simulink model "w3_warplab_trigger_proc"  (Simulink 7.7)
settings: Solver=ode45  StartTime=0.0  StopTime=60  RelTol=1e-3
InitFcn:
  | w3_warplab_trigger_proc_init
StartFcn:
  | w3_warplab_trigger_proc_init
undefined symbols (not defined in the file): gcbh, xlBlockLoadCallback, xlGetNormalizedPeriod
libraries: xbsIndex_r4 x1289, xbsEDKLib_r4 x1, simulink x1
(part 7 of 10)

== system w3_warplab_trigger_proc/Trigger Sources/CM PLL 2 ==
  Debounce Register{1..4} (4 alike) : xbsIndex_r4/Register  init=0  rst=off  en=off  dbl_ovrd=off  block_type=register
  Logical : xbsIndex_r4/Logical  logical_function=AND  inputs=4  en=off  latency=0  precision=Full  arith_type=Unsigned  n_bits=16  bin_pt=0  align_bp=on  dbl_ovrd=off  block_type=logical
  Mux : xbsIndex_r4/Mux  inputs=2  en=off  latency=0  precision=Full  arith_type=Unsigned  n_bits=16  bin_pt=14  quantization=Truncate  overflow=Wrap  dbl_ovrd=off  block_type=mux
  Trigger : Outport
  wires:
  Mux/1 -> Trigger/1
  Debounce Register1/1 -> Debounce Register2/1, Logical/1
  Debounce Register2/1 -> Debounce Register3/1, Logical/2
  Debounce Register3/1 -> Debounce Register4/1, Logical/3
  [Debug_2_Debounce] -> Mux/1
  Debounce Register4/1 -> Logical/4
  Logical/1 -> Mux/3
  [TRIG_DELAYED_CM_PLL_2] -> Mux/2, Debounce Register1/1

== system w3_warplab_trigger_proc/Trigger Sources/CM PLL 3 ==
  Debounce Register{1..4} (4 alike) : xbsIndex_r4/Register  init=0  rst=off  en=off  dbl_ovrd=off  block_type=register
  Logical : xbsIndex_r4/Logical  logical_function=AND  inputs=4  en=off  latency=0  precision=Full  arith_type=Unsigned  n_bits=16  bin_pt=0  align_bp=on  dbl_ovrd=off  block_type=logical
  Mux : xbsIndex_r4/Mux  inputs=2  en=off  latency=0  precision=Full  arith_type=Unsigned  n_bits=16  bin_pt=14  quantization=Truncate  overflow=Wrap  dbl_ovrd=off  block_type=mux
  Trigger : Outport
  wires:
  Logical/1 -> Mux/3
  Debounce Register4/1 -> Logical/4
  [Debug_3_Debounce] -> Mux/1
  Debounce Register3/1 -> Logical/3, Debounce Register4/1
  Debounce Register2/1 -> Logical/2, Debounce Register3/1
  Debounce Register1/1 -> Logical/1, Debounce Register2/1
  Mux/1 -> Trigger/1
  [TRIG_DELAYED_CM_PLL_3] -> Debounce Register1/1, Mux/2

== system w3_warplab_trigger_proc/Trigger Sources/Debug 0 ==
  Debounce Register{1..4} (4 alike) : xbsIndex_r4/Register  init=0  rst=off  en=off  dbl_ovrd=off  block_type=register
  Logical : xbsIndex_r4/Logical  logical_function=AND  inputs=4  en=off  latency=0  precision=Full  arith_type=Unsigned  n_bits=16  bin_pt=0  align_bp=on  dbl_ovrd=off  block_type=logical
  Mux : xbsIndex_r4/Mux  inputs=2  en=off  latency=0  precision=Full  arith_type=Unsigned  n_bits=16  bin_pt=14  quantization=Truncate  overflow=Wrap  dbl_ovrd=off  block_type=mux
  Trigger : Outport
  wires:
  Mux/1 -> Trigger/1
  Debounce Register1/1 -> Debounce Register2/1, Logical/1
  Debounce Register2/1 -> Logical/2, Debounce Register3/1
  Debounce Register3/1 -> Debounce Register4/1, Logical/3
  [Debug_0_Debounce] -> Mux/1
  Debounce Register4/1 -> Logical/4
  Logical/1 -> Mux/3
  [TRIG_DELAYED_DBG_HDR_0] -> Mux/2, Debounce Register1/1

== system w3_warplab_trigger_proc/Trigger Sources/Debug 1 ==
  Debounce Register{1..4} (4 alike) : xbsIndex_r4/Register  init=0  rst=off  en=off  dbl_ovrd=off  block_type=register
  Logical : xbsIndex_r4/Logical  logical_function=AND  inputs=4  en=off  latency=0  precision=Full  arith_type=Unsigned  n_bits=16  bin_pt=0  align_bp=on  dbl_ovrd=off  block_type=logical
  Mux : xbsIndex_r4/Mux  inputs=2  en=off  latency=0  precision=Full  arith_type=Unsigned  n_bits=16  bin_pt=14  quantization=Truncate  overflow=Wrap  dbl_ovrd=off  block_type=mux
  Trigger : Outport
  wires:
  Logical/1 -> Mux/3
  Debounce Register4/1 -> Logical/4
  [Debug_1_Debounce] -> Mux/1
  Debounce Register3/1 -> Logical/3, Debounce Register4/1
  Debounce Register2/1 -> Logical/2, Debounce Register3/1
  Debounce Register1/1 -> Logical/1, Debounce Register2/1
  Mux/1 -> Trigger/1
  [TRIG_DELAYED_DBG_HDR_1] -> Debounce Register1/1, Mux/2

== system w3_warplab_trigger_proc/Trigger Sources/Debug 2 ==
  Debounce Register{1..4} (4 alike) : xbsIndex_r4/Register  init=0  rst=off  en=off  dbl_ovrd=off  block_type=register
  Logical : xbsIndex_r4/Logical  logical_function=AND  inputs=4  en=off  latency=0  precision=Full  arith_type=Unsigned  n_bits=16  bin_pt=0  align_bp=on  dbl_ovrd=off  block_type=logical
  Mux : xbsIndex_r4/Mux  inputs=2  en=off  latency=0  precision=Full  arith_type=Unsigned  n_bits=16  bin_pt=14  quantization=Truncate  overflow=Wrap  dbl_ovrd=off  block_type=mux
  Trigger : Outport
  wires:
  Mux/1 -> Trigger/1
  Debounce Register1/1 -> Debounce Register2/1, Logical/1
  Debounce Register2/1 -> Debounce Register3/1, Logical/2
  Debounce Register3/1 -> Debounce Register4/1, Logical/3
  [Debug_2_Debounce] -> Mux/1
  Debounce Register4/1 -> Logical/4
  Logical/1 -> Mux/3
  [TRIG_DELAYED_DBG_HDR_2] -> Mux/2, Debounce Register1/1

== system w3_warplab_trigger_proc/Trigger Sources/Debug 3 ==
  Debounce Register{1..4} (4 alike) : xbsIndex_r4/Register  init=0  rst=off  en=off  dbl_ovrd=off  block_type=register
  Logical : xbsIndex_r4/Logical  logical_function=AND  inputs=4  en=off  latency=0  precision=Full  arith_type=Unsigned  n_bits=16  bin_pt=0  align_bp=on  dbl_ovrd=off  block_type=logical
  Mux : xbsIndex_r4/Mux  inputs=2  en=off  latency=0  precision=Full  arith_type=Unsigned  n_bits=16  bin_pt=14  quantization=Truncate  overflow=Wrap  dbl_ovrd=off  block_type=mux
  Trigger : Outport
  wires:
  Logical/1 -> Mux/3
  Debounce Register4/1 -> Logical/4
  [Debug_3_Debounce] -> Mux/1
  Debounce Register3/1 -> Logical/3, Debounce Register4/1
  Debounce Register2/1 -> Logical/2, Debounce Register3/1
  Debounce Register1/1 -> Logical/1, Debounce Register2/1
  Mux/1 -> Trigger/1
  [TRIG_DELAYED_DBG_HDR_3] -> Debounce Register1/1, Mux/2

== system w3_warplab_trigger_proc/Trigger Sources/Energy ==
  16LSB : xbsIndex_r4/Slice  nbits=16  boolean_output=off  mode=Lower Bit Location + Width  bit1=0  base1=MSB of Input  bit0=0  base0=LSB of Input  dbl_ovrd=off  block_type=slice
  16MSB : xbsIndex_r4/Slice  nbits=16  boolean_output=off  mode=Lower Bit Location + Width  bit1=0  base1=MSB of Input  bit0=16  base0=LSB of Input  dbl_ovrd=off  block_type=slice
  AntA Detector : Subsystem
  AntB Detector : Subsystem
  AntC Detector : Subsystem
  AntD Detector : Subsystem
  Convert : xbsIndex_r4/Convert  gui_display_data_type=Boolean  arith_type=Boolean  n_bits=16  bin_pt=14  float_type=Single  exp_bits=8  fraction_bits=24  quantization=Truncate  overflow=Wrap  en=off  latency=0  dbl_ovrd=off  pipeline=off  block_type=convert
  Display : Display
      settings: Format=hex (Stored Integer)
  Display1 : Display
      settings: Format=hex (Stored Integer)
  Display2 : Display
      settings: Format=hex (Stored Integer)
  Gateway Out1 : xbsIndex_r4/Gateway Out  inherit_from_input=off  hdl_port=off  timing_constraint=None  locs_specified=off  LOCs={}  UseAsDAC=off  DACChannel='1'  block_type=gatewayout
  Gateway Out2 : xbsIndex_r4/Gateway Out  inherit_from_input=off  hdl_port=off  timing_constraint=None  locs_specified=off  LOCs={}  UseAsDAC=off  DACChannel='1'  block_type=gatewayout
  Gateway Out6 : xbsIndex_r4/Gateway Out  inherit_from_input=off  hdl_port=off  timing_constraint=None  locs_specified=off  LOCs={}  UseAsDAC=off  DACChannel='1'  block_type=gatewayout
  MIMO Logic : Subsystem
  Posedge : Subsystem
  Pulse Generator : DiscretePulseGenerator  PulseType=Time based  Period=16  PulseWidth=50
  RFA_RSSI : xbsIndex_r4/Gateway In  gui_display_data_type=Fixed-point  arith_type=Unsigned  n_bits=10  bin_pt=0  preci_type=Single  exp_width=8  frac_width=24  quantization=Truncate  overflow=Wrap  period=1  dbl_ovrd=off  timing_constraint=None  locs_specified=off  LOCs={}  UseAsADC=off  ADCChannel='1'  inherit_from_input=off  hdl_port=on  block_type=gatewayin
      settings: block_version=VER_STRING_GOES_HERE
  RFB_RSSI : xbsIndex_r4/Gateway In  gui_display_data_type=Fixed-point  arith_type=Unsigned  n_bits=10  bin_pt=0  preci_type=Single  exp_width=8  frac_width=24  quantization=Truncate  overflow=Wrap  period=1  dbl_ovrd=off  timing_constraint=None  locs_specified=off  LOCs={}  UseAsADC=off  ADCChannel='1'  inherit_from_input=off  hdl_port=on  block_type=gatewayin
      settings: infoedit="Gateway in block.  Converts inputs of type Simulink integer, double and fixed point to  Xilinx fixed point type.<P><P>Hardware notes:  In hardware these blocks become top level input ports."  block_version=VER_STRING_GOES_HERE
  RFC_RSSI : xbsIndex_r4/Gateway In  gui_display_data_type=Fixed-point  arith_type=Unsigned  n_bits=10  bin_pt=0  preci_type=Single  exp_width=8  frac_width=24  quantization=Truncate  overflow=Wrap  period=1  dbl_ovrd=off  timing_constraint=None  locs_specified=off  LOCs={}  UseAsADC=off  ADCChannel='1'  inherit_from_input=off  hdl_port=on  block_type=gatewayin
      settings: infoedit="Gateway in block.  Converts inputs of type Simulink integer, double and fixed point to  Xilinx fixed point type.<P><P>Hardware notes:  In hardware these blocks become top level input ports."  block_version=VER_STRING_GOES_HERE
  RFD_RSSI : xbsIndex_r4/Gateway In  gui_display_data_type=Fixed-point  arith_type=Unsigned  n_bits=10  bin_pt=0  preci_type=Single  exp_width=8  frac_width=24  quantization=Truncate  overflow=Wrap  period=1  dbl_ovrd=off  timing_constraint=None  locs_specified=off  LOCs={}  UseAsADC=off  ADCChannel='1'  inherit_from_input=off  hdl_port=on  block_type=gatewayin
      settings: infoedit="Gateway in block.  Converts inputs of type Simulink integer, double and fixed point to  Xilinx fixed point type.<P><P>Hardware notes:  In hardware these blocks become top level input ports."  block_version=VER_STRING_GOES_HERE
  RSSI_CLK : xbsIndex_r4/Gateway In  gui_display_data_type=Boolean  arith_type=Boolean  n_bits=10  bin_pt=0  preci_type=Single  exp_width=8  frac_width=24  quantization=Truncate  overflow=Wrap  period=1  dbl_ovrd=off  timing_constraint=None  locs_specified=off  LOCs={}  UseAsADC=off  ADCChannel='1'  inherit_from_input=off  hdl_port=on  block_type=gatewayin
      settings: block_version=VER_STRING_GOES_HERE
  Repeating Sequence : simulink/Sources/Repeating Sequence  SystemSampleTime=-1  rep_seq_t=[0 200 600]  rep_seq_y=[0 1023 0]
  b0 : xbsIndex_r4/Slice  nbits=1  boolean_output=off  mode=Lower Bit Location + Width  bit1=0  base1=MSB of Input  bit0=0  base0=LSB of Input  dbl_ovrd=off  block_type=slice
  b1 : xbsIndex_r4/Slice  nbits=1  boolean_output=off  mode=Lower Bit Location + Width  bit1=0  base1=MSB of Input  bit0=1  base0=LSB of Input  dbl_ovrd=off  block_type=slice
  b2 : xbsIndex_r4/Slice  nbits=1  boolean_output=off  mode=Lower Bit Location + Width  bit1=0  base1=MSB of Input  bit0=2  base0=LSB of Input  dbl_ovrd=off  block_type=slice
  b3 : xbsIndex_r4/Slice  nbits=1  boolean_output=off  mode=Lower Bit Location + Width  bit1=0  base1=MSB of Input  bit0=3  base0=LSB of Input  dbl_ovrd=off  block_type=slice
  b31 : xbsIndex_r4/Slice  nbits=1  boolean_output=off  mode=Lower Bit Location + Width  bit1=0  base1=MSB of Input  bit0=31  base0=LSB of Input  dbl_ovrd=off  block_type=slice
  b[15:8] : xbsIndex_r4/Slice  nbits=8  boolean_output=off  mode=Lower Bit Location + Width  bit1=0  base1=MSB of Input  bit0=8  base0=LSB of Input  dbl_ovrd=off  block_type=slice
  b[20:16] : xbsIndex_r4/Slice  nbits=5  boolean_output=off  mode=Lower Bit Location + Width  bit1=0  base1=MSB of Input  bit0=16  base0=LSB of Input  dbl_ovrd=off  block_type=slice
  b[7:0] : xbsIndex_r4/Slice  nbits=8  boolean_output=off  mode=Lower Bit Location + Width  bit1=0  base1=MSB of Input  bit0=0  base0=LSB of Input  dbl_ovrd=off  block_type=slice
  Trigger : Outport
  tag scope: pktDetMask_A=global, pktDetMask_B=global, pktDetMask_C=global, pktDetMask_D=global, pktDetReset=global, pktDet_duration_busy=global, pktDet_duration_idle=global, pktDet_energyThresh_busy=global, pktDet_energyThresh_idle=global, regPktDet_RSSIavgLength=global
  wires:
  AntA Detector/1(pktdet) -> MIMO Logic/1(Det A)
  [pktDetReset] -> Convert/1
  RFA_RSSI/1 -> AntA Detector/1(RSSI)
  [reg_pkt_det_config] -> b0/1, b1/1, b2/1, b3/1, Gateway Out6/1, b31/1
  [reg_pkt_det_thresh] -> 16LSB/1, 16MSB/1, Gateway Out1/1
  [reg_pkt_det_duration] -> b[7:0]/1, b[15:8]/1, b[20:16]/1, Gateway Out2/1
  16LSB/1 -> [pktDet_energyThresh_idle]
  16MSB/1 -> [pktDet_energyThresh_busy]
  b[7:0]/1 -> [pktDet_duration_idle]
  b[15:8]/1 -> [pktDet_duration_busy]
  b[20:16]/1 -> [regPktDet_RSSIavgLength]
  AntB Detector/1(pktdet) -> MIMO Logic/2(Det B)
  AntC Detector/1(pktdet) -> MIMO Logic/3(Det C)
  AntD Detector/1(pktdet) -> MIMO Logic/4(Det D)
  RFB_RSSI/1 -> AntB Detector/1(RSSI)
  RFC_RSSI/1 -> AntC Detector/1(RSSI)
  RFD_RSSI/1 -> AntD Detector/1(RSSI)
  Convert/1 -> AntA Detector/2(Reset), AntB Detector/2(Reset), AntC Detector/2(Reset), AntD Detector/2(Reset)
  MIMO Logic/1(PktDet) -> Trigger/1
  RSSI_CLK/1 -> Posedge/1(D)
  Posedge/1(Q) -> AntC Detector/3(En), AntD Detector/3(En), AntB Detector/3(En), AntA Detector/3(En)
  Repeating Sequence/1 -> RFA_RSSI/1, RFB_RSSI/1, RFC_RSSI/1, RFD_RSSI/1
  Pulse Generator/1 -> RSSI_CLK/1
  Gateway Out6/1 -> Display/1
  Gateway Out1/1 -> Display1/1
  Gateway Out2/1 -> Display2/1
  b0/1 -> [pktDetMask_A]
  b1/1 -> [pktDetMask_B]
  b2/1 -> [pktDetMask_C]
  b3/1 -> [pktDetMask_D]
  b31/1 -> [pktDetReset]

== system w3_warplab_trigger_proc/Trigger Sources/Ethernet A ==
  Constant{,1..4,6..7} (7 alike) : Constant  Value=0
  ETH_A_AXI_STR_TDATA : xbsIndex_r4/Gateway In  gui_display_data_type=Fixed-point  arith_type=Unsigned  n_bits=32  bin_pt=0  preci_type=Single  exp_width=8  frac_width=24  quantization="Round  (unbiased: +/- Inf)"  overflow=Wrap  period=1  dbl_ovrd=off  timing_constraint=None  locs_specified=off  LOCs={}  UseAsADC=off  ADCChannel='1'  inherit_from_input=off  hdl_port=on  block_type=gatewayin
  ETH_A_AXI_STR_TDEST : xbsIndex_r4/Gateway In  gui_display_data_type=Fixed-point  arith_type=Unsigned  n_bits=4  bin_pt=0  preci_type=Single  exp_width=8  frac_width=24  quantization="Round  (unbiased: +/- Inf)"  overflow=Wrap  period=1  dbl_ovrd=off  timing_constraint=None  locs_specified=off  LOCs={}  UseAsADC=off  ADCChannel='1'  inherit_from_input=off  hdl_port=on  block_type=gatewayin
  ETH_A_AXI_STR_TKEEP : xbsIndex_r4/Gateway In  gui_display_data_type=Fixed-point  arith_type=Unsigned  n_bits=4  bin_pt=0  preci_type=Single  exp_width=8  frac_width=24  quantization="Round  (unbiased: +/- Inf)"  overflow=Wrap  period=1  dbl_ovrd=off  timing_constraint=None  locs_specified=off  LOCs={}  UseAsADC=off  ADCChannel='1'  inherit_from_input=off  hdl_port=on  block_type=gatewayin
  ETH_A_AXI_STR_TLAST : xbsIndex_r4/Gateway In  gui_display_data_type=Fixed-point  arith_type=Unsigned  n_bits=1  bin_pt=0  preci_type=Single  exp_width=8  frac_width=24  quantization="Round  (unbiased: +/- Inf)"  overflow=Wrap  period=1  dbl_ovrd=off  timing_constraint=None  locs_specified=off  LOCs={}  UseAsADC=off  ADCChannel='1'  inherit_from_input=off  hdl_port=on  block_type=gatewayin
  ETH_A_AXI_STR_TREADY : xbsIndex_r4/Gateway In  gui_display_data_type=Fixed-point  arith_type=Unsigned  n_bits=1  bin_pt=0  preci_type=Single  exp_width=8  frac_width=24  quantization="Round  (unbiased: +/- Inf)"  overflow=Wrap  period=1  dbl_ovrd=off  timing_constraint=None  locs_specified=off  LOCs={}  UseAsADC=off  ADCChannel='1'  inherit_from_input=off  hdl_port=on  block_type=gatewayin
  ETH_A_AXI_STR_TSTRB : xbsIndex_r4/Gateway In  gui_display_data_type=Fixed-point  arith_type=Unsigned  n_bits=4  bin_pt=0  preci_type=Single  exp_width=8  frac_width=24  quantization="Round  (unbiased: +/- Inf)"  overflow=Wrap  period=1  dbl_ovrd=off  timing_constraint=None  locs_specified=off  LOCs={}  UseAsADC=off  ADCChannel='1'  inherit_from_input=off  hdl_port=on  block_type=gatewayin
  ETH_A_AXI_STR_TVALID : xbsIndex_r4/Gateway In  gui_display_data_type=Fixed-point  arith_type=Unsigned  n_bits=1  bin_pt=0  preci_type=Single  exp_width=8  frac_width=24  quantization="Round  (unbiased: +/- Inf)"  overflow=Wrap  period=1  dbl_ovrd=off  timing_constraint=None  locs_specified=off  LOCs={}  UseAsADC=off  ADCChannel='1'  inherit_from_input=off  hdl_port=on  block_type=gatewayin
  HW_SW_Select : xbsIndex_r4/Mux  inputs=2  en=off  latency=0  precision=Full  arith_type=Unsigned  n_bits=16  bin_pt=14  quantization=Truncate  overflow=Wrap  dbl_ovrd=off  block_type=mux
  Pkt Comp : Subsystem
  Terminator : Terminator
  Terminator1 : Terminator
  Terminator2 : Terminator
  Trigger : Outport
  wires:
  Constant/1 -> ETH_A_AXI_STR_TVALID/1
  Constant1/1 -> ETH_A_AXI_STR_TDATA/1
  Constant2/1 -> ETH_A_AXI_STR_TLAST/1
  Constant3/1 -> ETH_A_AXI_STR_TSTRB/1
  ETH_A_AXI_STR_TVALID/1 -> Pkt Comp/1(TVALID)  "TVALID"
  ETH_A_AXI_STR_TDATA/1 -> Pkt Comp/2(TDATA)  "TDATA"
  ETH_A_AXI_STR_TREADY/1 -> Pkt Comp/3(TREADY)  "TREADY"
  Constant4/1 -> ETH_A_AXI_STR_TREADY/1
  ETH_A_AXI_STR_TLAST/1 -> Pkt Comp/4(TLAST)  "TLAST"
  Constant6/1 -> ETH_A_AXI_STR_TKEEP/1
  Constant7/1 -> ETH_A_AXI_STR_TDEST/1
  ETH_A_AXI_STR_TDEST/1 -> Terminator2/1  "TDEST"
  ETH_A_AXI_STR_TKEEP/1 -> Terminator1/1  "TKEEP"
  ETH_A_AXI_STR_TSTRB/1 -> Terminator/1  "TSTRB"
  Pkt Comp/1(Trigger) -> HW_SW_Select/2
  [Eth_A_HW_SW_Sel] -> HW_SW_Select/1
  [Eth_A_SW_Trig] -> HW_SW_Select/3
  HW_SW_Select/1 -> Trigger/1

== system w3_warplab_trigger_proc/Trigger Sources/Ethernet B ==
  Constant{,1..4,6..7} (7 alike) : Constant  Value=0
  ETH_B_AXI_STR_TDATA : xbsIndex_r4/Gateway In  gui_display_data_type=Fixed-point  arith_type=Unsigned  n_bits=32  bin_pt=0  preci_type=Single  exp_width=8  frac_width=24  quantization="Round  (unbiased: +/- Inf)"  overflow=Wrap  period=1  dbl_ovrd=off  timing_constraint=None  locs_specified=off  LOCs={}  UseAsADC=off  ADCChannel='1'  inherit_from_input=off  hdl_port=on  block_type=gatewayin
  ETH_B_AXI_STR_TDEST : xbsIndex_r4/Gateway In  gui_display_data_type=Fixed-point  arith_type=Unsigned  n_bits=4  bin_pt=0  preci_type=Single  exp_width=8  frac_width=24  quantization="Round  (unbiased: +/- Inf)"  overflow=Wrap  period=1  dbl_ovrd=off  timing_constraint=None  locs_specified=off  LOCs={}  UseAsADC=off  ADCChannel='1'  inherit_from_input=off  hdl_port=on  block_type=gatewayin
  ETH_B_AXI_STR_TKEEP : xbsIndex_r4/Gateway In  gui_display_data_type=Fixed-point  arith_type=Unsigned  n_bits=4  bin_pt=0  preci_type=Single  exp_width=8  frac_width=24  quantization="Round  (unbiased: +/- Inf)"  overflow=Wrap  period=1  dbl_ovrd=off  timing_constraint=None  locs_specified=off  LOCs={}  UseAsADC=off  ADCChannel='1'  inherit_from_input=off  hdl_port=on  block_type=gatewayin
  ETH_B_AXI_STR_TLAST : xbsIndex_r4/Gateway In  gui_display_data_type=Fixed-point  arith_type=Unsigned  n_bits=1  bin_pt=0  preci_type=Single  exp_width=8  frac_width=24  quantization="Round  (unbiased: +/- Inf)"  overflow=Wrap  period=1  dbl_ovrd=off  timing_constraint=None  locs_specified=off  LOCs={}  UseAsADC=off  ADCChannel='1'  inherit_from_input=off  hdl_port=on  block_type=gatewayin
  ETH_B_AXI_STR_TREADY : xbsIndex_r4/Gateway In  gui_display_data_type=Fixed-point  arith_type=Unsigned  n_bits=1  bin_pt=0  preci_type=Single  exp_width=8  frac_width=24  quantization="Round  (unbiased: +/- Inf)"  overflow=Wrap  period=1  dbl_ovrd=off  timing_constraint=None  locs_specified=off  LOCs={}  UseAsADC=off  ADCChannel='1'  inherit_from_input=off  hdl_port=on  block_type=gatewayin
  ETH_B_AXI_STR_TSTRB : xbsIndex_r4/Gateway In  gui_display_data_type=Fixed-point  arith_type=Unsigned  n_bits=4  bin_pt=0  preci_type=Single  exp_width=8  frac_width=24  quantization="Round  (unbiased: +/- Inf)"  overflow=Wrap  period=1  dbl_ovrd=off  timing_constraint=None  locs_specified=off  LOCs={}  UseAsADC=off  ADCChannel='1'  inherit_from_input=off  hdl_port=on  block_type=gatewayin
  ETH_B_AXI_STR_TVALID : xbsIndex_r4/Gateway In  gui_display_data_type=Fixed-point  arith_type=Unsigned  n_bits=1  bin_pt=0  preci_type=Single  exp_width=8  frac_width=24  quantization="Round  (unbiased: +/- Inf)"  overflow=Wrap  period=1  dbl_ovrd=off  timing_constraint=None  locs_specified=off  LOCs={}  UseAsADC=off  ADCChannel='1'  inherit_from_input=off  hdl_port=on  block_type=gatewayin
  HW_SW_Select : xbsIndex_r4/Mux  inputs=2  en=off  latency=0  precision=Full  arith_type=Unsigned  n_bits=16  bin_pt=14  quantization=Truncate  overflow=Wrap  dbl_ovrd=off  block_type=mux
  Pkt Comp : Subsystem
  Terminator : Terminator
  Terminator1 : Terminator
  Terminator2 : Terminator
  Trigger : Outport
  wires:
  Constant/1 -> ETH_B_AXI_STR_TVALID/1
  Constant1/1 -> ETH_B_AXI_STR_TDATA/1
  Constant2/1 -> ETH_B_AXI_STR_TLAST/1
  Constant3/1 -> ETH_B_AXI_STR_TSTRB/1
  ETH_B_AXI_STR_TVALID/1 -> Pkt Comp/1(TVALID)  "TVALID"
  ETH_B_AXI_STR_TDATA/1 -> Pkt Comp/2(TDATA)  "TDATA"
  ETH_B_AXI_STR_TREADY/1 -> Pkt Comp/3(TREADY)  "TREADY"
  Constant4/1 -> ETH_B_AXI_STR_TREADY/1
  ETH_B_AXI_STR_TLAST/1 -> Pkt Comp/4(TLAST)  "TLAST"
  Constant6/1 -> ETH_B_AXI_STR_TKEEP/1
  Constant7/1 -> ETH_B_AXI_STR_TDEST/1
  ETH_B_AXI_STR_TDEST/1 -> Terminator2/1  "TDEST"
  ETH_B_AXI_STR_TKEEP/1 -> Terminator1/1  "TKEEP"
  ETH_B_AXI_STR_TSTRB/1 -> Terminator/1  "TSTRB"
  [Eth_B_HW_SW_Sel] -> HW_SW_Select/1
  [Eth_B_SW_Trig] -> HW_SW_Select/3
  Pkt Comp/1(Trigger) -> HW_SW_Select/2
  HW_SW_Select/1 -> Trigger/1

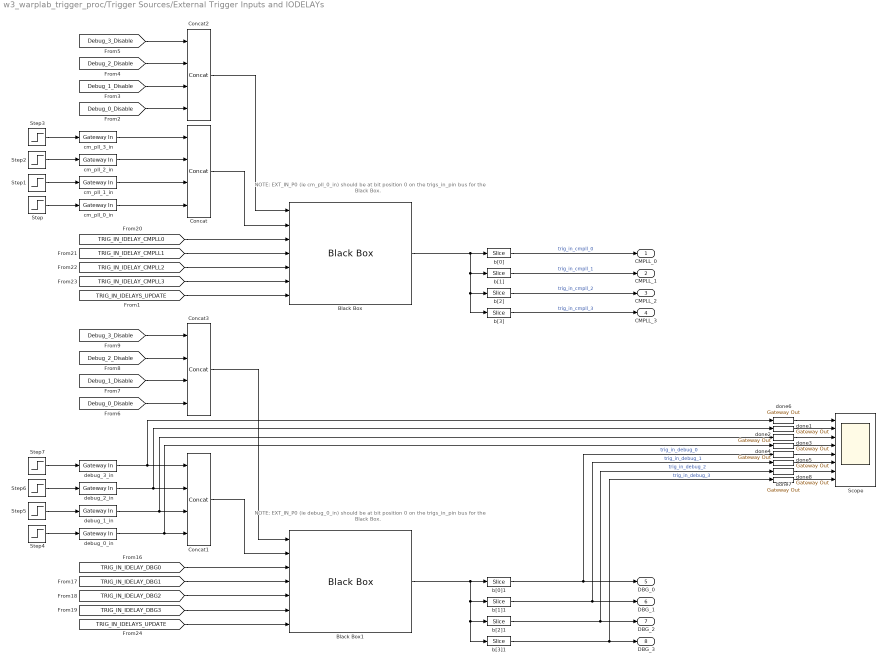
== system w3_warplab_trigger_proc/Trigger Sources/External Trigger Inputs and IODELAYs ==
  note: NOTE:  EXT_IN_P0 (ie cm_pll_0_in) should be at bit
      |         position 0 on the trigs_in_pin bus for the Black Box.
  note: NOTE:  EXT_IN_P0 (ie debug_0_in) should be at bit
      |         position 0 on the trigs_in_pin bus for the Black Box.
  Black Box : xbsIndex_r4/Black Box  init_code=trig_idelays_config  sim_method=ISE Simulator  verbose=off  block_type=blackbox2
  Black Box1 : xbsIndex_r4/Black Box  init_code=trig_idelays_config  sim_method=ISE Simulator  verbose=off  block_type=blackbox2
  Concat{,1..3} (4 alike) : xbsIndex_r4/Concat  num_inputs=4  dbl_ovrd=off  block_type=concat
  Scope : Scope  NumInputPorts=8
      settings: YMin=-5~-5~-5~-5~-5~-5~-5~-5  YMax=5~5~5~5~5~5~5~5  SaveName=ScopeData2
  Step{,1..3} (4 alike) : Step  Time=50  After=0  SampleTime=1
  Step{4..7} (4 alike) : Step  Time=50  SampleTime=1
  b[0] : xbsIndex_r4/Slice  nbits=1  boolean_output=off  mode=Lower Bit Location + Width  bit1=0  base1=MSB of Input  bit0=0  base0=LSB of Input  dbl_ovrd=off  block_type=slice
  b[0]1 : xbsIndex_r4/Slice  nbits=1  boolean_output=off  mode=Lower Bit Location + Width  bit1=0  base1=MSB of Input  bit0=0  base0=LSB of Input  dbl_ovrd=off  block_type=slice
  b[1] : xbsIndex_r4/Slice  nbits=1  boolean_output=off  mode=Lower Bit Location + Width  bit1=0  base1=MSB of Input  bit0=1  base0=LSB of Input  dbl_ovrd=off  block_type=slice
  b[1]1 : xbsIndex_r4/Slice  nbits=1  boolean_output=off  mode=Lower Bit Location + Width  bit1=0  base1=MSB of Input  bit0=1  base0=LSB of Input  dbl_ovrd=off  block_type=slice
  b[2] : xbsIndex_r4/Slice  nbits=1  boolean_output=off  mode=Lower Bit Location + Width  bit1=0  base1=MSB of Input  bit0=2  base0=LSB of Input  dbl_ovrd=off  block_type=slice
  b[2]1 : xbsIndex_r4/Slice  nbits=1  boolean_output=off  mode=Lower Bit Location + Width  bit1=0  base1=MSB of Input  bit0=2  base0=LSB of Input  dbl_ovrd=off  block_type=slice
  b[3] : xbsIndex_r4/Slice  nbits=1  boolean_output=off  mode=Lower Bit Location + Width  bit1=0  base1=MSB of Input  bit0=3  base0=LSB of Input  dbl_ovrd=off  block_type=slice
  b[3]1 : xbsIndex_r4/Slice  nbits=1  boolean_output=off  mode=Lower Bit Location + Width  bit1=0  base1=MSB of Input  bit0=3  base0=LSB of Input  dbl_ovrd=off  block_type=slice
  cm_pll_0_in : xbsIndex_r4/Gateway In  gui_display_data_type=Boolean  arith_type=Boolean  n_bits=16  bin_pt=14  preci_type=Single  exp_width=8  frac_width=24  quantization="Round  (unbiased: +/- Inf)"  overflow=Saturate  period=1  dbl_ovrd=off  timing_constraint=None  locs_specified=off  LOCs={}  UseAsADC=off  ADCChannel='1'  inherit_from_input=off  hdl_port=on  block_type=gatewayin
  cm_pll_1_in : xbsIndex_r4/Gateway In  gui_display_data_type=Boolean  arith_type=Boolean  n_bits=16  bin_pt=14  preci_type=Single  exp_width=8  frac_width=24  quantization="Round  (unbiased: +/- Inf)"  overflow=Saturate  period=1  dbl_ovrd=off  timing_constraint=None  locs_specified=off  LOCs={}  UseAsADC=off  ADCChannel='1'  inherit_from_input=off  hdl_port=on  block_type=gatewayin
  cm_pll_2_in : xbsIndex_r4/Gateway In  gui_display_data_type=Boolean  arith_type=Boolean  n_bits=16  bin_pt=14  preci_type=Single  exp_width=8  frac_width=24  quantization="Round  (unbiased: +/- Inf)"  overflow=Saturate  period=1  dbl_ovrd=off  timing_constraint=None  locs_specified=off  LOCs={}  UseAsADC=off  ADCChannel='1'  inherit_from_input=off  hdl_port=on  block_type=gatewayin
  cm_pll_3_in : xbsIndex_r4/Gateway In  gui_display_data_type=Boolean  arith_type=Boolean  n_bits=16  bin_pt=14  preci_type=Single  exp_width=8  frac_width=24  quantization="Round  (unbiased: +/- Inf)"  overflow=Saturate  period=1  dbl_ovrd=off  timing_constraint=None  locs_specified=off  LOCs={}  UseAsADC=off  ADCChannel='1'  inherit_from_input=off  hdl_port=on  block_type=gatewayin
  debug_0_in : xbsIndex_r4/Gateway In  gui_display_data_type=Boolean  arith_type=Boolean  n_bits=16  bin_pt=14  preci_type=Single  exp_width=8  frac_width=24  quantization="Round  (unbiased: +/- Inf)"  overflow=Saturate  period=1  dbl_ovrd=off  timing_constraint=None  locs_specified=off  LOCs={}  UseAsADC=off  ADCChannel='1'  inherit_from_input=off  hdl_port=on  block_type=gatewayin
  debug_1_in : xbsIndex_r4/Gateway In  gui_display_data_type=Boolean  arith_type=Boolean  n_bits=16  bin_pt=14  preci_type=Single  exp_width=8  frac_width=24  quantization="Round  (unbiased: +/- Inf)"  overflow=Saturate  period=1  dbl_ovrd=off  timing_constraint=None  locs_specified=off  LOCs={}  UseAsADC=off  ADCChannel='1'  inherit_from_input=off  hdl_port=on  block_type=gatewayin
  debug_2_in : xbsIndex_r4/Gateway In  gui_display_data_type=Boolean  arith_type=Boolean  n_bits=16  bin_pt=14  preci_type=Single  exp_width=8  frac_width=24  quantization="Round  (unbiased: +/- Inf)"  overflow=Saturate  period=1  dbl_ovrd=off  timing_constraint=None  locs_specified=off  LOCs={}  UseAsADC=off  ADCChannel='1'  inherit_from_input=off  hdl_port=on  block_type=gatewayin
  debug_3_in : xbsIndex_r4/Gateway In  gui_display_data_type=Boolean  arith_type=Boolean  n_bits=16  bin_pt=14  preci_type=Single  exp_width=8  frac_width=24  quantization="Round  (unbiased: +/- Inf)"  overflow=Saturate  period=1  dbl_ovrd=off  timing_constraint=None  locs_specified=off  LOCs={}  UseAsADC=off  ADCChannel='1'  inherit_from_input=off  hdl_port=on  block_type=gatewayin
  done{1..8} (8 alike) : xbsIndex_r4/Gateway Out  inherit_from_input=off  hdl_port=off  timing_constraint=None  locs_specified=off  LOCs={}  UseAsDAC=off  DACChannel='1'  block_type=gatewayout
      settings: infoedit="Gateway out block.  Converts Xilinx fixed point inputs into ouputs of type Simulink integer, double, or fixed point.<P><P>Hardware notes:  In hardware these blocks become top level output ports or are discarded, depending on how they are configured."  xl_area=[0 0 0 0 1 0 0]  block_version=VER_STRING_GOES_HERE
  CMPLL_0 : Outport
  CMPLL_1 : Outport  Port=2
  CMPLL_2 : Outport  Port=3
  CMPLL_3 : Outport  Port=4
  DBG_0 : Outport  Port=5
  DBG_1 : Outport  Port=6
  DBG_2 : Outport  Port=7
  DBG_3 : Outport  Port=8
  wires:
  Step/1 -> cm_pll_0_in/1
  Step1/1 -> cm_pll_1_in/1
  Step2/1 -> cm_pll_2_in/1
  Step3/1 -> cm_pll_3_in/1
  Step4/1 -> debug_0_in/1
  Step5/1 -> debug_1_in/1
  Step6/1 -> debug_2_in/1
  Step7/1 -> debug_3_in/1
  Black Box/1 -> b[0]/1, b[1]/1, b[2]/1, b[3]/1
  Black Box1/1 -> b[3]1/1, b[2]1/1, b[1]1/1, b[0]1/1
  b[0]/1 -> CMPLL_0/1  "trig_in_cmpll_0"
  b[1]/1 -> CMPLL_1/1  "trig_in_cmpll_1"
  b[2]/1 -> CMPLL_2/1  "trig_in_cmpll_2"
  b[3]/1 -> CMPLL_3/1  "trig_in_cmpll_3"
  b[0]1/1 -> DBG_0/1, done4/1  "trig_in_debug_0"
  b[1]1/1 -> DBG_1/1, done5/1  "trig_in_debug_1"
  b[2]1/1 -> DBG_2/1, done7/1  "trig_in_debug_2"
  b[3]1/1 -> DBG_3/1, done8/1  "trig_in_debug_3"
  cm_pll_3_in/1 -> Concat/1
  cm_pll_2_in/1 -> Concat/2
  cm_pll_1_in/1 -> Concat/3
  cm_pll_0_in/1 -> Concat/4
  debug_3_in/1 -> Concat1/1, done6/1
  debug_2_in/1 -> Concat1/2, done1/1
  debug_1_in/1 -> Concat1/3, done2/1
  debug_0_in/1 -> Concat1/4, done3/1
  done6/1 -> Scope/1
  done1/1 -> Scope/2
  done2/1 -> Scope/3
  done3/1 -> Scope/4
  done4/1 -> Scope/5
  done5/1 -> Scope/6
  done7/1 -> Scope/7
  done8/1 -> Scope/8
  [TRIG_IN_IDELAYS_UPDATE] -> Black Box/7
  Concat/1 -> Black Box/2
  [TRIG_IN_IDELAY_CMPLL0] -> Black Box/3
  [TRIG_IN_IDELAY_CMPLL1] -> Black Box/4
  [TRIG_IN_IDELAY_CMPLL2] -> Black Box/5
  [TRIG_IN_IDELAY_CMPLL3] -> Black Box/6
  Concat1/1 -> Black Box1/2
  [TRIG_IN_IDELAY_DBG0] -> Black Box1/3
  [TRIG_IN_IDELAY_DBG1] -> Black Box1/4
  [TRIG_IN_IDELAY_DBG2] -> Black Box1/5
  [TRIG_IN_IDELAY_DBG3] -> Black Box1/6
  [TRIG_IN_IDELAYS_UPDATE] -> Black Box1/7
  [Debug_3_Disable] -> Concat2/1
  [Debug_2_Disable] -> Concat2/2
  [Debug_1_Disable] -> Concat2/3
  [Debug_0_Disable] -> Concat2/4
  Concat2/1 -> Black Box/1
  [Debug_3_Disable] -> Concat3/1
  [Debug_2_Disable] -> Concat3/2
  [Debug_1_Disable] -> Concat3/3
  [Debug_0_Disable] -> Concat3/4
  Concat3/1 -> Black Box1/1

== system w3_warplab_trigger_proc/Trigger Sources/Software ==
  Trigger : Outport
  wires:
  [Software_Trig] -> Trigger/1

== system w3_warplab_trigger_proc/Trigger Sources/Energy/AntA Detector ==
  RSSI : Inport
  Reset : Inport  Port=2
  En : Inport  Port=3
  ASR : xbsIndex_r4/Addressable Shift Register  infer_latency=on  depth=2  initVector=[0]  en=on  dbl_ovrd=off  use_behavioral_HDL=off  Optimization=Resource  use_rpm=off  block_type=addrsr
      settings: infoedit="Delay of configurable length.  Any element in the delay line can be addressed and driven onto the output port.<br><br>Hardware notes: This block is implemented using SRL16s. If Virtex-4 or Spartan-3 device is used, multiple SRLC16s are cascaded together."  block_version=VER_STRING_GOES_HERE
  Busy Detection : Subsystem
  Delay : xbsIndex_r4/Delay  rst=off  infoeditControl=Selection of Reset will increase slice count due to use of real FFs and instead of SRLs  en=off  latency=2  dbl_ovrd=off  reg_retiming=off  block_type=delay
  Display : Display
  Gateway Out{,1..6} (7 alike) : xbsIndex_r4/Gateway Out  inherit_from_input=off  hdl_port=off  timing_constraint=None  locs_specified=off  LOCs={}  UseAsDAC=off  DACChannel='1'  block_type=gatewayout
      Gateway Out settings: infoedit="Gateway out block.  Converts Xilinx fixed point inputs into ouputs of type Simulink integer, double, or fixed point.<P><P>Hardware notes:  In hardware these blocks become top level output ports or are discarded, depending on how they are configured."  block_version=8.2
      Gateway Out1 settings: infoedit="Gateway out block.  Converts Xilinx fixed point inputs into ouputs of type Simulink integer, double, or fixed point.<P><P>Hardware notes:  In hardware these blocks become top level output ports or are discarded, depending on how they are configured."  block_version=8.2
      Gateway Out2 settings: infoedit="Gateway out block.  Converts Xilinx fixed point inputs into ouputs of type Simulink integer, double, or fixed point.<P><P>Hardware notes:  In hardware these blocks become top level output ports or are discarded, depending on how they are configured."  block_version=8.2
      Gateway Out3 settings: infoedit="Gateway out block.  Converts Xilinx fixed point inputs into ouputs of type Simulink integer, double, or fixed point.<P><P>Hardware notes:  In hardware these blocks become top level output ports or are discarded, depending on how they are configured."  block_version=8.2
      Gateway Out4 settings: infoedit="Gateway out block.  Converts Xilinx fixed point inputs into ouputs of type Simulink integer, double, or fixed point.<P><P>Hardware notes:  In hardware these blocks become top level output ports or are discarded, depending on how they are configured."  block_version=8.2
      Gateway Out5 settings: infoedit="Gateway out block.  Converts Xilinx fixed point inputs into ouputs of type Simulink integer, double, or fixed point.<P><P>Hardware notes:  In hardware these blocks become top level output ports or are discarded, depending on how they are configured."  block_version=8.2
  Idle Detection : Subsystem
  Logical : xbsIndex_r4/Logical  logical_function=AND  inputs=2  en=off  latency=0  precision=Full  arith_type=Unsigned  n_bits=16  bin_pt=0  align_bp=on  dbl_ovrd=off  block_type=logical
  Pkt Det Decision : Scope  NumInputPorts=6
      settings: TimeRange=1000  YMin=0~0~0~0~0~0  YMax=1000~15000~1~1~1~1
  Running Sum : Subsystem
  pktdet : Outport
  wires:
  Reset/1 -> Running Sum/2(reset), Idle Detection/2(Reset), Busy Detection/2(Reset)
  [regPktDet_RSSIavgLength] -> Running Sum/3(avglen), Gateway Out6/1
  Gateway Out/1 -> Pkt Det Decision/1  "RAWRSSI"
  Gateway Out1/1 -> Pkt Det Decision/2  "AVGRSSI"
  Gateway Out2/1 -> Pkt Det Decision/3  "IDLE"
  RSSI/1 -> Running Sum/1(RSSI), Gateway Out/1
  Running Sum/1(avg) -> Idle Detection/1(Avg RSSI), Busy Detection/1(Avg RSSI), Gateway Out1/1
  Idle Detection/1(Idle) -> Gateway Out2/1, Delay/1
  [pktDet_duration_busy] -> ASR/2
  ASR/1 -> Logical/1, Gateway Out5/1
  Busy Detection/1(Busy) -> Logical/2, Gateway Out3/1
  Logical/1 -> pktdet/1, Gateway Out4/1
  Gateway Out3/1 -> Pkt Det Decision/5  "BUSY"
  Gateway Out4/1 -> Pkt Det Decision/6  "DET"
  Gateway Out5/1 -> Pkt Det Decision/4  "IDLE DLY"
  Delay/1 -> ASR/1
  En/1 -> Running Sum/4(en), ASR/3, Idle Detection/3(en), Busy Detection/3(en)
  Gateway Out6/1 -> Display/1

== system w3_warplab_trigger_proc/Trigger Sources/Energy/AntB Detector ==
  RSSI : Inport
  Reset : Inport  Port=2
  En : Inport  Port=3
  ASR : xbsIndex_r4/Addressable Shift Register  infer_latency=on  depth=2  initVector=[0]  en=on  dbl_ovrd=off  use_behavioral_HDL=off  Optimization=Resource  use_rpm=off  block_type=addrsr
      settings: infoedit="Delay of configurable length.  Any element in the delay line can be addressed and driven onto the output port.<br><br>Hardware notes: This block is implemented using SRL16s. If Virtex-4 or Spartan-3 device is used, multiple SRLC16s are cascaded together."  block_version=VER_STRING_GOES_HERE
  Busy Detection : Subsystem
  Delay : xbsIndex_r4/Delay  rst=off  infoeditControl=Selection of Reset will increase slice count due to use of real FFs and instead of SRLs  en=off  latency=2  dbl_ovrd=off  reg_retiming=off  block_type=delay
  Gateway Out{,1..5} (6 alike) : xbsIndex_r4/Gateway Out  inherit_from_input=off  hdl_port=off  timing_constraint=None  locs_specified=off  LOCs={}  UseAsDAC=off  DACChannel='1'  block_type=gatewayout
      settings: infoedit="Gateway out block.  Converts Xilinx fixed point inputs into ouputs of type Simulink integer, double, or fixed point.<P><P>Hardware notes:  In hardware these blocks become top level output ports or are discarded, depending on how they are configured."  block_version=8.2
  Idle Detection : Subsystem
  Logical : xbsIndex_r4/Logical  logical_function=AND  inputs=2  en=off  latency=0  precision=Full  arith_type=Unsigned  n_bits=16  bin_pt=0  align_bp=on  dbl_ovrd=off  block_type=logical
  Pkt Det Decision : Scope  NumInputPorts=6
      settings: TimeRange=1000  YMin=0~0~0~0~0~0  YMax=1000~15000~1~1~1~1
  Running Sum : Subsystem
  pktdet : Outport
  wires:
  En/1 -> ASR/3, Idle Detection/3(en), Busy Detection/3(en), Running Sum/4(en)
  Delay/1 -> ASR/1
  Gateway Out5/1 -> Pkt Det Decision/4  "IDLE DLY"
  Gateway Out4/1 -> Pkt Det Decision/6  "DET"
  Gateway Out3/1 -> Pkt Det Decision/5  "BUSY"
  Logical/1 -> Gateway Out4/1, pktdet/1
  Busy Detection/1(Busy) -> Gateway Out3/1, Logical/2
  ASR/1 -> Gateway Out5/1, Logical/1
  [pktDet_duration_busy] -> ASR/2
  Idle Detection/1(Idle) -> Delay/1, Gateway Out2/1
  Running Sum/1(avg) -> Gateway Out1/1, Idle Detection/1(Avg RSSI), Busy Detection/1(Avg RSSI)
  RSSI/1 -> Gateway Out/1, Running Sum/1(RSSI)
  Gateway Out2/1 -> Pkt Det Decision/3  "IDLE"
  Gateway Out1/1 -> Pkt Det Decision/2  "AVGRSSI"
  Gateway Out/1 -> Pkt Det Decision/1  "RAWRSSI"
  [regPktDet_RSSIavgLength] -> Running Sum/3(avglen)
  Reset/1 -> Idle Detection/2(Reset), Busy Detection/2(Reset), Running Sum/2(reset)

== system w3_warplab_trigger_proc/Trigger Sources/Energy/AntC Detector ==
  RSSI : Inport
  Reset : Inport  Port=2
  En : Inport  Port=3
  ASR : xbsIndex_r4/Addressable Shift Register  infer_latency=on  depth=2  initVector=[0]  en=on  dbl_ovrd=off  use_behavioral_HDL=off  Optimization=Resource  use_rpm=off  block_type=addrsr
      settings: infoedit="Delay of configurable length.  Any element in the delay line can be addressed and driven onto the output port.<br><br>Hardware notes: This block is implemented using SRL16s. If Virtex-4 or Spartan-3 device is used, multiple SRLC16s are cascaded together."  block_version=VER_STRING_GOES_HERE
  Busy Detection : Subsystem
  Delay : xbsIndex_r4/Delay  rst=off  infoeditControl=Selection of Reset will increase slice count due to use of real FFs and instead of SRLs  en=off  latency=2  dbl_ovrd=off  reg_retiming=off  block_type=delay
  Gateway Out{,1..5} (6 alike) : xbsIndex_r4/Gateway Out  inherit_from_input=off  hdl_port=off  timing_constraint=None  locs_specified=off  LOCs={}  UseAsDAC=off  DACChannel='1'  block_type=gatewayout
      settings: infoedit="Gateway out block.  Converts Xilinx fixed point inputs into ouputs of type Simulink integer, double, or fixed point.<P><P>Hardware notes:  In hardware these blocks become top level output ports or are discarded, depending on how they are configured."  block_version=8.2
  Idle Detection : Subsystem
  Logical : xbsIndex_r4/Logical  logical_function=AND  inputs=2  en=off  latency=0  precision=Full  arith_type=Unsigned  n_bits=16  bin_pt=0  align_bp=on  dbl_ovrd=off  block_type=logical
  Pkt Det Decision : Scope  NumInputPorts=6
      settings: TimeRange=1000  YMin=0~0~0~0~0~0  YMax=1000~15000~1~1~1~1
  Running Sum : Subsystem
  pktdet : Outport
  wires:
  Reset/1 -> Running Sum/2(reset), Busy Detection/2(Reset), Idle Detection/2(Reset)
  [regPktDet_RSSIavgLength] -> Running Sum/3(avglen)
  Gateway Out/1 -> Pkt Det Decision/1  "RAWRSSI"
  Gateway Out1/1 -> Pkt Det Decision/2  "AVGRSSI"
  Gateway Out2/1 -> Pkt Det Decision/3  "IDLE"
  RSSI/1 -> Running Sum/1(RSSI), Gateway Out/1
  Running Sum/1(avg) -> Busy Detection/1(Avg RSSI), Idle Detection/1(Avg RSSI), Gateway Out1/1
  Idle Detection/1(Idle) -> Gateway Out2/1, Delay/1
  [pktDet_duration_busy] -> ASR/2
  ASR/1 -> Logical/1, Gateway Out5/1
  Busy Detection/1(Busy) -> Logical/2, Gateway Out3/1
  Logical/1 -> pktdet/1, Gateway Out4/1
  Gateway Out3/1 -> Pkt Det Decision/5  "BUSY"
  Gateway Out4/1 -> Pkt Det Decision/6  "DET"
  Gateway Out5/1 -> Pkt Det Decision/4  "IDLE DLY"
  Delay/1 -> ASR/1
  En/1 -> Running Sum/4(en), ASR/3, Busy Detection/3(en), Idle Detection/3(en)

== system w3_warplab_trigger_proc/Trigger Sources/Energy/AntD Detector ==
  RSSI : Inport
  Reset : Inport  Port=2
  En : Inport  Port=3
  ASR : xbsIndex_r4/Addressable Shift Register  infer_latency=on  depth=2  initVector=[0]  en=on  dbl_ovrd=off  use_behavioral_HDL=off  Optimization=Resource  use_rpm=off  block_type=addrsr
      settings: infoedit="Delay of configurable length.  Any element in the delay line can be addressed and driven onto the output port.<br><br>Hardware notes: This block is implemented using SRL16s. If Virtex-4 or Spartan-3 device is used, multiple SRLC16s are cascaded together."  block_version=VER_STRING_GOES_HERE
  Busy Detection : Subsystem
  Delay : xbsIndex_r4/Delay  rst=off  infoeditControl=Selection of Reset will increase slice count due to use of real FFs and instead of SRLs  en=off  latency=2  dbl_ovrd=off  reg_retiming=off  block_type=delay
  Gateway Out{,1..5} (6 alike) : xbsIndex_r4/Gateway Out  inherit_from_input=off  hdl_port=off  timing_constraint=None  locs_specified=off  LOCs={}  UseAsDAC=off  DACChannel='1'  block_type=gatewayout
      settings: infoedit="Gateway out block.  Converts Xilinx fixed point inputs into ouputs of type Simulink integer, double, or fixed point.<P><P>Hardware notes:  In hardware these blocks become top level output ports or are discarded, depending on how they are configured."  block_version=8.2
  Idle Detection : Subsystem
  Logical : xbsIndex_r4/Logical  logical_function=AND  inputs=2  en=off  latency=0  precision=Full  arith_type=Unsigned  n_bits=16  bin_pt=0  align_bp=on  dbl_ovrd=off  block_type=logical
  Pkt Det Decision : Scope  NumInputPorts=6
      settings: TimeRange=1000  YMin=0~0~0~0~0~0  YMax=1000~15000~1~1~1~1
  Running Sum : Subsystem
  pktdet : Outport
  wires:
  En/1 -> ASR/3, Idle Detection/3(en), Busy Detection/3(en), Running Sum/4(en)
  Delay/1 -> ASR/1
  Gateway Out5/1 -> Pkt Det Decision/4  "IDLE DLY"
  Gateway Out4/1 -> Pkt Det Decision/6  "DET"
  Gateway Out3/1 -> Pkt Det Decision/5  "BUSY"
  Logical/1 -> Gateway Out4/1, pktdet/1
  Busy Detection/1(Busy) -> Gateway Out3/1, Logical/2
  ASR/1 -> Gateway Out5/1, Logical/1
  [pktDet_duration_busy] -> ASR/2
  Idle Detection/1(Idle) -> Delay/1, Gateway Out2/1
  Running Sum/1(avg) -> Gateway Out1/1, Idle Detection/1(Avg RSSI), Busy Detection/1(Avg RSSI)
  RSSI/1 -> Gateway Out/1, Running Sum/1(RSSI)
  Gateway Out2/1 -> Pkt Det Decision/3  "IDLE"
  Gateway Out1/1 -> Pkt Det Decision/2  "AVGRSSI"
  Gateway Out/1 -> Pkt Det Decision/1  "RAWRSSI"
  [regPktDet_RSSIavgLength] -> Running Sum/3(avglen)
  Reset/1 -> Idle Detection/2(Reset), Busy Detection/2(Reset), Running Sum/2(reset)

== system w3_warplab_trigger_proc/Trigger Sources/Energy/MIMO Logic ==
  Det A : Inport
  Det B : Inport  Port=2
  Det C : Inport  Port=3
  Det D : Inport  Port=4
  Convert{1..8} (8 alike) : xbsIndex_r4/Convert  gui_display_data_type=Fixed-point  arith_type=Unsigned  n_bits=1  bin_pt=0  float_type=Single  exp_bits=8  fraction_bits=24  quantization=Truncate  overflow=Flag as error  en=off  latency=0  dbl_ovrd=off  pipeline=off  block_type=convert
      settings: block_version=10.1.3
  Logical{,1,3..4} (4 alike) : xbsIndex_r4/Logical  logical_function=AND  inputs=2  en=off  latency=0  precision=Full  arith_type=Unsigned  n_bits=16  bin_pt=0  align_bp=on  dbl_ovrd=off  block_type=logical
  Logical2 : xbsIndex_r4/Logical  logical_function=OR  inputs=4  en=off  latency=0  precision=Full  arith_type=Unsigned  n_bits=16  bin_pt=0  align_bp=on  dbl_ovrd=off  block_type=logical
  PktDet : Outport
  wires:
  [pktDetMask_A] -> Convert2/1
  [pktDetMask_B] -> Convert3/1
  Det A/1 -> Convert7/1
  Det B/1 -> Convert1/1
  Convert7/1 -> Logical/1
  Convert2/1 -> Logical/2
  Convert1/1 -> Logical1/1
  Convert3/1 -> Logical1/2
  Logical/1 -> Logical2/1
  Logical1/1 -> Logical2/2
  Logical2/1 -> PktDet/1
  [pktDetMask_C] -> Convert5/1
  Det C/1 -> Convert4/1
  Convert4/1 -> Logical3/1
  Convert5/1 -> Logical3/2
  Logical3/1 -> Logical2/3
  [pktDetMask_D] -> Convert8/1
  Det D/1 -> Convert6/1
  Convert6/1 -> Logical4/1
  Convert8/1 -> Logical4/2
  Logical4/1 -> Logical2/4

== system w3_warplab_trigger_proc/Trigger Sources/Energy/Posedge ==
  D : Inport
  Delay : xbsIndex_r4/Delay  rst=off  infoeditControl=Selection of Reset will increase slice count due to use of real FFs and instead of SRLs  en=off  latency=1  dbl_ovrd=off  reg_retiming=off  block_type=delay
      settings: infoedit=Hardware notes: A delay line is a chain, each link of which is an SRL16 followed by a flip-flop. If register retiming is enabled, the delay line is a chain of flip-flops.  block_version=8.2
  Inverter : xbsIndex_r4/Inverter  en=off  latency=0  dbl_ovrd=off  block_type=inv
      settings: block_version=8.2
  Logical : xbsIndex_r4/Logical  logical_function=AND  inputs=2  en=off  latency=0  precision=Full  arith_type=Unsigned  n_bits=16  bin_pt=0  align_bp=on  dbl_ovrd=off  block_type=logical
      settings: block_version=8.2
  Q : Outport
  wires:
  D/1 -> Inverter/1, Logical/1
  Inverter/1 -> Delay/1
  Delay/1 -> Logical/2
  Logical/1 -> Q/1

== system w3_warplab_trigger_proc/Trigger Sources/Ethernet A/Pkt Comp ==
  TVALID : Inport
  TDATA : Inport  Port=2
  TREADY : Inport  Port=3
  TLAST : Inport  Port=4
  Convert2 : xbsIndex_r4/Convert  gui_display_data_type=Boolean  arith_type=Boolean  n_bits=16  bin_pt=14  float_type=Single  exp_bits=8  fraction_bits=24  quantization=Truncate  overflow=Wrap  en=off  latency=0  dbl_ovrd=off  pipeline=off  block_type=convert
  Convert3 : xbsIndex_r4/Convert  gui_display_data_type=Boolean  arith_type=Boolean  n_bits=16  bin_pt=14  float_type=Single  exp_bits=8  fraction_bits=24  quantization=Truncate  overflow=Wrap  en=off  latency=0  dbl_ovrd=off  pipeline=off  block_type=convert
  Delay : xbsIndex_r4/Delay  rst=off  infoeditControl=Selection of Reset will increase slice count due to use of real FFs and instead of SRLs  en=off  latency=4  dbl_ovrd=off  reg_retiming=off  block_type=delay
  Delay1 : xbsIndex_r4/Delay  rst=off  infoeditControl=Selection of Reset will increase slice count due to use of real FFs and instead of SRLs  en=off  latency=3  dbl_ovrd=off  reg_retiming=off  block_type=delay
  Delay2 : xbsIndex_r4/Delay  rst=off  infoeditControl=Selection of Reset will increase slice count due to use of real FFs and instead of SRLs  en=off  latency=1  dbl_ovrd=off  reg_retiming=off  block_type=delay
  Delay3 : xbsIndex_r4/Delay  rst=off  infoeditControl=Selection of Reset will increase slice count due to use of real FFs and instead of SRLs  en=off  latency=1  dbl_ovrd=off  reg_retiming=off  block_type=delay
  Logical : xbsIndex_r4/Logical  logical_function=AND  inputs=2  en=off  latency=0  precision=Full  arith_type=Unsigned  n_bits=16  bin_pt=0  align_bp=on  dbl_ovrd=off  block_type=logical
  Output Reg 0 : Subsystem
  Pkt Match 0 : Subsystem
  Pkt Word Addr : xbsIndex_r4/Counter  cnt_type=Count Limited  cnt_to=63  operation=Up  start_count=0  cnt_by_val=1  arith_type=Unsigned  n_bits=6  bin_pt=0  load_pin=off  rst=on  en=on  explicit_period=off  period=1  dbl_ovrd=off  use_behavioral_HDL=off  implementation=Fabric  block_type=counter
  Register : xbsIndex_r4/Register  init=0  rst=off  en=off  dbl_ovrd=off  block_type=register
  Register1 : xbsIndex_r4/Register  init=0  rst=off  en=off  dbl_ovrd=off  block_type=register
  Register2 : xbsIndex_r4/Register  init=0  rst=off  en=off  dbl_ovrd=off  block_type=register
  Word Comp 0 : Subsystem
  Trigger : Outport
  wires:
  Logical/1 -> Convert2/1
  TVALID/1 -> Logical/1
  TREADY/1 -> Logical/2
  Pkt Word Addr/1 -> Word Comp 0/1(Word Addr)
  TLAST/1 -> Convert3/1
  Convert2/1 -> Pkt Word Addr/2, Delay3/1
  Convert3/1 -> Pkt Word Addr/1, Delay/1, Delay1/1
  TDATA/1 -> Delay2/1
  Delay/1 -> Register1/1
  Word Comp 0/1(Word Match) -> Pkt Match 0/2(Word Match)
  Delay1/1 -> Register2/1
  Pkt Match 0/1(Pkt Match) -> Output Reg 0/1(Match)
  Output Reg 0/1(Out) -> Trigger/1
  Delay2/1 -> Word Comp 0/2(TDATA)
  Delay3/1 -> Register/1
  Register/1 -> Pkt Match 0/1(Valid)
  Register1/1 -> Pkt Match 0/3(Reset)
  Register2/1 -> Output Reg 0/2(Done)
